simulink model "Equipe9_Simulateur_Matlab"  (R2023a)
settings: Solver=ode45  StartTime=0.0  StopTime=temps  RelTol=1e-7  EnableMultiTasking=on
model workspace (MAT data in the model file):
  K = 0.745
  K_2 = 0.745
  K_3 = 0.854
  T = 146.07
  T_2 = 38.431
  T_3 = 20.268
values from neighbouring files (symbols this model uses):
  ampli_diff = 3.075    [interface.m]
  B = 3984    [interface.m]
  bit_adc = 10    [interface.m]
  bit_dac = 10    [interface.m]
  courant_finale = 1    [interface.m]
  courant_initiale = 0    [interface.m]
  courant_timer = 10    [interface.m]
  Cte_filtre = 0.00944    [interface.m]
  Cte_perturbation = 150.4664    [interface.m]
  Cte_perturbationT2 = 150.3737    [interface.m]
  Cte_T1 = 90.126    [interface.m]
  Cte_T2 = 38.431    [interface.m]
  Cte_T3 = 20.268    [interface.m]
  final_temps = temps    (= 1000)    [interface.m]
  finalPower = 0    [interface.m]
  finalTemp = 25    [interface.m]
  Gain_circuit_sortie = 0.24801    [interface.m]
  Gain_perturbation = 6.1526    [interface.m]
  Gain_perturbationT2 = 5.5789    [interface.m]
  Gain_puissance = 3.2071    [interface.m]
  Gain_T1 = 8.192    [interface.m]
  Gain_T2 = 0.745    [interface.m]
  Gain_T3 = 0.854    [interface.m]
  gainReg = 0.1    [interface.m]
  initialPower = 0    [interface.m]
  initialTemp = 23    [interface.m]
  initialTime = 0    [interface.m]
  plus_petite = 1.735    [interface.m]
  ProportionT2 = 1    [interface.m]
  R_0 = 10000    [interface.m]
  samplingTime = 3    [interface.m]
  T_0 = 298.15    [interface.m]
  tempsReg = 130    [interface.m]
  V_ref = 2.521    [interface.m]
  variance = 0.0025    [interface.m]
undefined symbols (not defined in the file or in its folder): boucleouverte, pwm_ouvert, samplingTimePWM
libraries: eePwmGenerator x1
settings Model: Creator=LiberT  LastModifiedBy=SAPAR95
settings SolverCC: AlgebraicLoopSolver=TrustRegion
settings DataIOCC: LimitDataPoints=on  SaveFormat=Array  SignalLoggingSaveFormat=ModelDataLogs  ReturnWorkspaceOutputs=off
settings OptimizationCC: BlockReduction=off  BooleanDataType=off  OptimizeBlockIOStorage=off  ExpressionDepthLimit=2147483647  InitFltsAndDblsToZero=on  LifeSpan=inf
settings DebuggingCC: SaveWithParameterizedLinksMsg=none  UnderspecifiedInitializationDetection=Classic  MergeDetectMultiDrivingBlocksExec=none  SignalResolutionControl=TryResolveAllWithWarning  MultiTaskDSMMsg=warning  MultiTaskCondExecSysMsg=none  FcnCallInpInsideContextMsg=warning  UnconnectedInputMsg=warning  UnconnectedOutputMsg=warning  UnconnectedLineMsg=warning  StateNameClashWarn=warning  SFUnexpectedBacktrackingDiag=warning  SFNoUnconditionalDefaultTransitionDiag=warning  SFExecutionAtInitializationDiag=none  ArithmeticOperatorsInVariantConditions=warning
settings HardwareCC: ProdBitPerPointer=32  ProdBitPerSizeT=32  ProdBitPerPtrDiffT=32  ProdLargestAtomicFloat=None  ProdIntDivRoundTo=Undefined  ProdEndianess=Unspecified  ProdWordSize=32  ProdHWDeviceType=32-bit Generic  TargetBitPerPointer=64  TargetBitPerSizeT=64  TargetBitPerPtrDiffT=64  TargetLongLongMode=on  TargetIntDivRoundTo=Zero  TargetEndianess=LittleEndian  TargetWordSize=64  TargetHWDeviceType=MATLAB Host  ProdEqTarget=off
settings ModelReferenceCC: EnableRefExpFcnMdlSchedulingChecks=on  PropagateSignalLabelsOutOfModel=off
settings SFSimCC: SimUseLocalCustomCode=off  CustomCodeUndefinedFunction=UseInterfaceOnly
settings RTWCC: RTWUseLocalCustomCode=off
settings CodeAppCC: StateflowObjectComments=on
settings GRTTargetCC: TargetFcnLib=ansi_tfl_tmw.mat  TargetLangStandard=C89/C90 (ANSI)  ModelReferenceCompliant=off  CompOptLevelCompliant=off  CombineOutputUpdateFcns=off  MatFileLogging=off  GRTInterface=on
settings ConfigComp: CovMetricSettings=dw  CovSaveCumulativeToWorkspaceVar=on  CovSaveSingleToWorkspaceVar=on  CovExternalEMLEnable=off

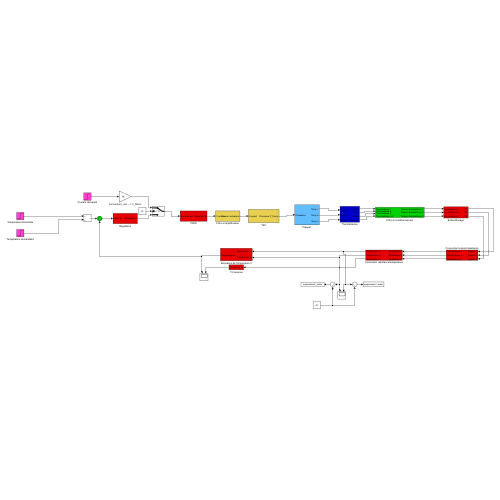
[thumbnail: Simulink's stored preview of the top-level diagram]
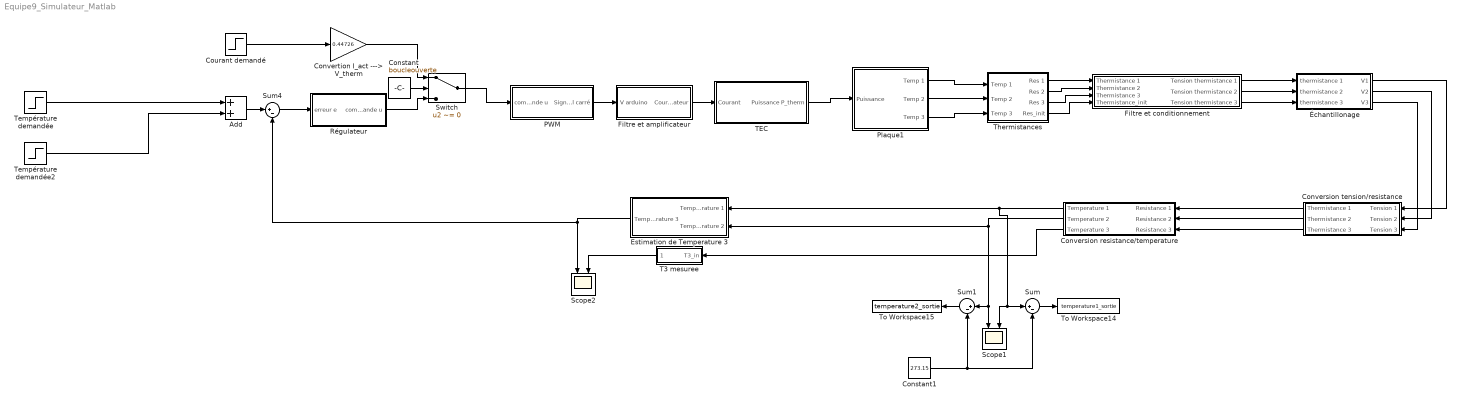
== system Equipe9_Simulateur_Matlab ==
  Add : Sum
  Constant : Constant  Value=boucleouverte
  Constant1 : Constant  Value=273.15
  Conversion resistance/temperature : Subsystem
  Conversion tension/resistance : Subsystem
  Convertion I_act ---> V_therm : Gain  Gain=0.44726
  Courant demandé : Step  Time=courant_timer  Before=courant_initiale  After=courant_finale  SampleTime=0
  Estimation de Temperature 3 : Subsystem
  Filtre et amplificateur : Subsystem
  Filtre et conditionnement : Subsystem
  PWM : Subsystem
  Plaque1 : Subsystem
  Régulateur : Subsystem
  Scope1 : Scope  NumInputPorts=2
  Scope2 : Scope  NumInputPorts=2
  Sum : Sum  Inputs=|+-
  Sum1 : Sum  Inputs=|+-
  Sum4 : Sum  Inputs=|+-  InputSameDT=on  SaturateOnIntegerOverflow=on  OutDataTypeStr=Inherit: Same as first input
  Switch : Switch  Criteria=u2 ~= 0  Threshold=false  SaturateOnIntegerOverflow=off  InputSameDT=off
  T3 mesuree : Subsystem
  TEC : Subsystem
  Température demandée : Step  Time=0  Before=initialTemp  After=finalTemp  SampleTime=0
  Température demandée2 : Step  Time=final_temps  After=final_final-finalTemp  SampleTime=0
  Thermistances : Subsystem
  To Workspace14 : ToWorkspace  VariableName=temperature1_sortie  SaveFormat=Timeseries  SampleTime=samplingTime
  To Workspace15 : ToWorkspace  VariableName=temperature2_sortie  SaveFormat=Timeseries  SampleTime=samplingTime
  Échantillonage : Subsystem
  wires:
  Sum4/1 -> Régulateur/1(erreur e)
  Plaque1/3(Temp 3) -> Thermistances/3(Temp 3)
  Filtre et amplificateur/1(Courant actuateur) -> TEC/1(Courant)
  Plaque1/1(Temp 1) -> Thermistances/1(Temp 1)
  Plaque1/2(Temp 2) -> Thermistances/2(Temp 2)
  Filtre et conditionnement/1(Tension thermistance 1) -> Échantillonage/1(thermistance 1)
  Conversion tension/resistance/2(Thermistance 2) -> Conversion resistance/temperature/2(Resistance 2)
  Conversion resistance/temperature/1(Temperature 1) -> Sum/1, Scope1/2, Estimation de Temperature 3/1(Temperature 1)
  Conversion resistance/temperature/2(Temperature 2) -> Sum1/1, Scope1/1, Estimation de Temperature 3/2(Temperature 2)
  Estimation de Temperature 3/1(Temperature 3) -> Scope2/1, Sum4/2
  PWM/1(Signal carré) -> Filtre et amplificateur/1(V arduino)
  Thermistances/3(Res 3) -> Filtre et conditionnement/3(Thermistance 3)
  Thermistances/2(Res 2) -> Filtre et conditionnement/2(Thermistance 2)
  T3 mesuree/1(T3_out) -> Scope2/2
  Conversion resistance/temperature/3(Temperature 3) -> T3 mesuree/1(T3_in)
  Filtre et conditionnement/3(Tension thermistance 3) -> Échantillonage/3(thermistance 3)
  Échantillonage/1(V1) -> Conversion tension/resistance/1(Tension 1)
  Échantillonage/2(V2) -> Conversion tension/resistance/2(Tension 2)
  Échantillonage/3(V3) -> Conversion tension/resistance/3(Tension 3)
  Régulateur/1(commande u) -> Switch/3
  Switch/1 -> PWM/1(commande u)
  Constant/1 -> Switch/2
  Courant demandé/1 -> Convertion I_act ---> V_therm/1
  Convertion I_act ---> V_therm/1 -> Switch/1
  Thermistances/1(Res 1) -> Filtre et conditionnement/1(Thermistance 1)
  Conversion tension/resistance/3(Thermistance 3) -> Conversion resistance/temperature/3(Resistance 3)
  Conversion tension/resistance/1(Thermistance 1) -> Conversion resistance/temperature/1(Resistance 1)
  Filtre et conditionnement/2(Tension thermistance 2) -> Échantillonage/2(thermistance 2)
  TEC/1(Puissance P_therm) -> Plaque1/1(Puissance)
  Thermistances/4(Res_init) -> Filtre et conditionnement/4(Thermistance_init)
  Température demandée/1 -> Add/1
  Température demandée2/1 -> Add/2
  Add/1 -> Sum4/1
  Sum/1 -> To Workspace14/1
  Constant1/1 -> Sum1/2, Sum/2
  Sum1/1 -> To Workspace15/1

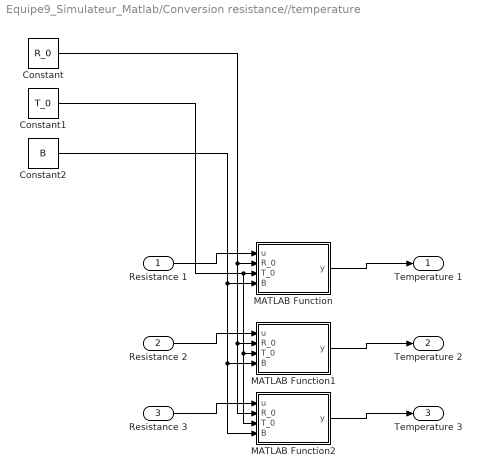
== system Equipe9_Simulateur_Matlab/Conversion resistance//temperature ==
  Resistance 1 : Inport
  Resistance 2 : Inport  Port=2
  Resistance 3 : Inport  Port=3
  Constant : Constant  Value=R_0
  Constant1 : Constant  Value=T_0
  Constant2 : Constant  Value=B
  MATLAB Function : MATLAB Function  TreatAsAtomicUnit=on
  MATLAB Function1 : MATLAB Function  TreatAsAtomicUnit=on
  MATLAB Function2 : MATLAB Function  TreatAsAtomicUnit=on
  Temperature 1 : Outport
  Temperature 2 : Outport  Port=2
  Temperature 3 : Outport  Port=3
  wires:
  Resistance 1/1 -> MATLAB Function/1(u)
  MATLAB Function/1(y) -> Temperature 1/1
  Resistance 2/1 -> MATLAB Function1/1(u)
  MATLAB Function1/1(y) -> Temperature 2/1
  Resistance 3/1 -> MATLAB Function2/1(u)
  MATLAB Function2/1(y) -> Temperature 3/1
  Constant/1 -> MATLAB Function2/2(R_0), MATLAB Function1/2(R_0), MATLAB Function/2(R_0)
  Constant1/1 -> MATLAB Function2/3(T_0), MATLAB Function1/3(T_0), MATLAB Function/3(T_0)
  Constant2/1 -> MATLAB Function/4(B), MATLAB Function1/4(B), MATLAB Function2/4(B)

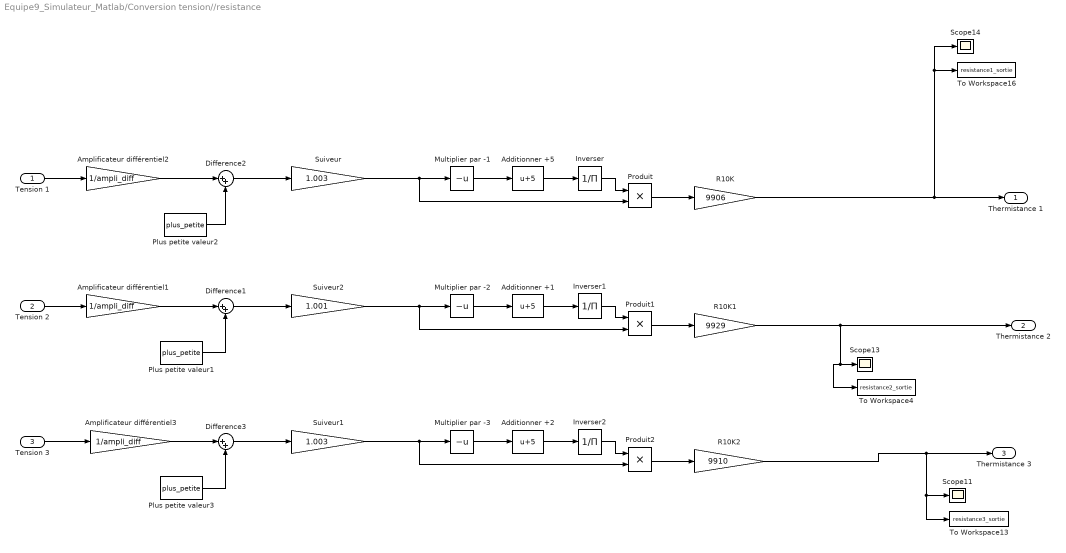
== system Equipe9_Simulateur_Matlab/Conversion tension//resistance ==
  Tension 1 : Inport
  Tension 2 : Inport  Port=2
  Tension 3 : Inport  Port=3
  Additionner +1 : Bias  Bias=5  SaturateOnIntegerOverflow=off
  Additionner +2 : Bias  Bias=5  SaturateOnIntegerOverflow=off
  Additionner +5 : Bias  Bias=5  SaturateOnIntegerOverflow=off
  Amplificateur différentiel1 : Gain  Gain=1/ampli_diff
  Amplificateur différentiel2 : Gain  Gain=1/ampli_diff
  Amplificateur différentiel3 : Gain  Gain=1/ampli_diff
  Difference1 : Sum  Inputs=|++
  Difference2 : Sum  Inputs=|++
  Difference3 : Sum  Inputs=|++
  Inverser : Product  Inputs=/
  Inverser1 : Product  Inputs=/
  Inverser2 : Product  Inputs=/
  Multiplier par -1 : UnaryMinus
  Multiplier par -2 : UnaryMinus
  Multiplier par -3 : UnaryMinus
  Plus petite valeur1 : Constant  Value=plus_petite
  Plus petite valeur2 : Constant  Value=plus_petite
  Plus petite valeur3 : Constant  Value=plus_petite
  Produit : Product
  Produit1 : Product
  Produit2 : Product
  R10K : Gain  Gain=9906
  R10K1 : Gain  Gain=9929
  R10K2 : Gain  Gain=9910
  Scope11 : Scope
  Scope13 : Scope
  Scope14 : Scope
  Suiveur : Gain  Gain=1.003
  Suiveur1 : Gain  Gain=1.003
  Suiveur2 : Gain  Gain=1.001
  To Workspace13 : ToWorkspace  VariableName=resistance3_sortie  SaveFormat=Timeseries  SampleTime=samplingTime
  To Workspace16 : ToWorkspace  VariableName=resistance1_sortie  SaveFormat=Timeseries  SampleTime=samplingTime
  To Workspace4 : ToWorkspace  VariableName=resistance2_sortie  SaveFormat=Timeseries  SampleTime=samplingTime
  Thermistance 1 : Outport
  Thermistance 2 : Outport  Port=2
  Thermistance 3 : Outport  Port=3
  wires:
  Difference2/1 -> Suiveur/1
  Inverser/1 -> Produit/1
  Multiplier par -1/1 -> Additionner +5/1
  Produit/1 -> R10K/1
  Additionner +5/1 -> Inverser/1
  Amplificateur différentiel2/1 -> Difference2/1
  Plus petite valeur2/1 -> Difference2/2
  Tension 1/1 -> Amplificateur différentiel2/1
  Plus petite valeur1/1 -> Difference1/2
  Difference1/1 -> Suiveur2/1
  Produit1/1 -> R10K1/1
  Tension 2/1 -> Amplificateur différentiel1/1
  Amplificateur différentiel1/1 -> Difference1/1
  Multiplier par -2/1 -> Additionner +1/1
  Inverser1/1 -> Produit1/1
  Additionner +1/1 -> Inverser1/1
  Additionner +2/1 -> Inverser2/1
  Multiplier par -3/1 -> Additionner +2/1
  Amplificateur différentiel3/1 -> Difference3/1
  Plus petite valeur3/1 -> Difference3/2
  Inverser2/1 -> Produit2/1
  Difference3/1 -> Suiveur1/1
  Tension 3/1 -> Amplificateur différentiel3/1
  Produit2/1 -> R10K2/1
  Suiveur/1 -> Produit/2, Multiplier par -1/1
  Suiveur1/1 -> Produit2/2, Multiplier par -3/1
  Suiveur2/1 -> Produit1/2, Multiplier par -2/1
  R10K/1 -> Scope14/1, To Workspace16/1, Thermistance 1/1
  R10K1/1 -> To Workspace4/1, Scope13/1, Thermistance 2/1
  R10K2/1 -> To Workspace13/1, Scope11/1, Thermistance 3/1

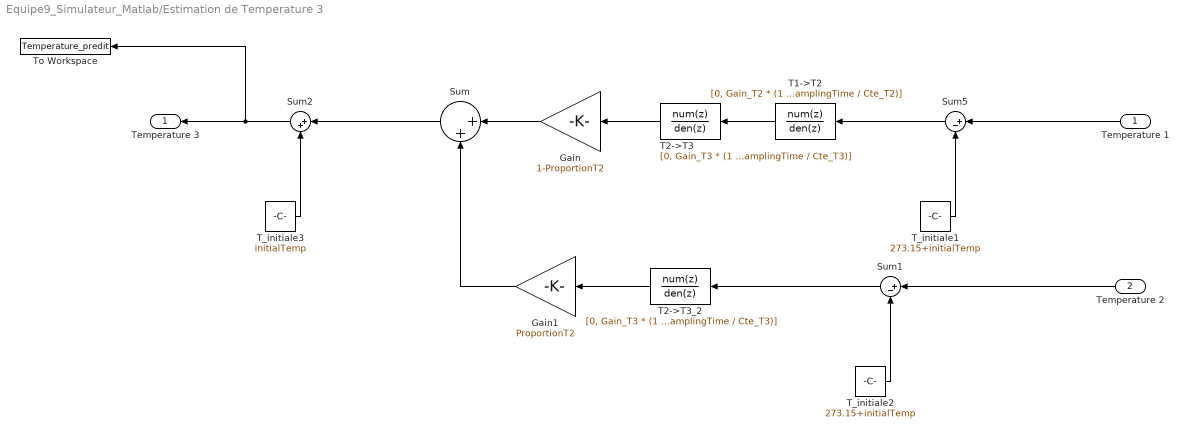
== system Equipe9_Simulateur_Matlab/Estimation de Temperature 3 ==
  Temperature 1 : Inport
  Temperature 2 : Inport  Port=2
  Gain : Gain  Gain=1-ProportionT2
  Gain1 : Gain  Gain=ProportionT2
  Sum : Sum  Inputs=|++
  Sum1 : Sum  Inputs=|+-  InputSameDT=on  SaturateOnIntegerOverflow=on  OutDataTypeStr=Inherit: Same as first input
  Sum2 : Sum  Inputs=|++  InputSameDT=on  SaturateOnIntegerOverflow=on  OutDataTypeStr=Inherit: Same as first input
  Sum5 : Sum  Inputs=|+-  InputSameDT=on  SaturateOnIntegerOverflow=on  OutDataTypeStr=Inherit: Same as first input
  T1->T2 : DiscreteFilter  Numerator=[0, Gain_T2 * (1 - exp(-samplingTime / Cte_T2))]  Denominator=[1, -exp(-samplingTime / Cte_T2)]  SampleTime=samplingTime
  T2->T3 : DiscreteFilter  Numerator=[0, Gain_T3 * (1 - exp(-samplingTime / Cte_T3))]  Denominator=[1, -exp(-samplingTime / Cte_T3)]  SampleTime=samplingTime
  T2->T3_2 : DiscreteFilter  Numerator=[0, Gain_T3 * (1 - exp(-samplingTime / Cte_T3))]  Denominator=[1, -exp(-samplingTime / Cte_T3)]  SampleTime=samplingTime
  T_initiale1 : Constant  Value=273.15+initialTemp
  T_initiale2 : Constant  Value=273.15+initialTemp
  T_initiale3 : Constant  Value=initialTemp
  To Workspace : ToWorkspace  VariableName=Temperature_predit  SaveFormat=Timeseries  SampleTime=samplingTime
  Temperature 3 : Outport
  wires:
  Temperature 2/1 -> Sum1/1
  T_initiale2/1 -> Sum1/2
  T_initiale3/1 -> Sum2/2
  Sum1/1 -> T2->T3_2/1
  T1->T2/1 -> T2->T3/1
  T2->T3/1 -> Gain/1
  Sum5/1 -> T1->T2/1
  Temperature 1/1 -> Sum5/1
  T_initiale1/1 -> Sum5/2
  Sum/1 -> Sum2/1
  T2->T3_2/1 -> Gain1/1
  Gain/1 -> Sum/1
  Gain1/1 -> Sum/2
  Sum2/1 -> To Workspace/1, Temperature 3/1

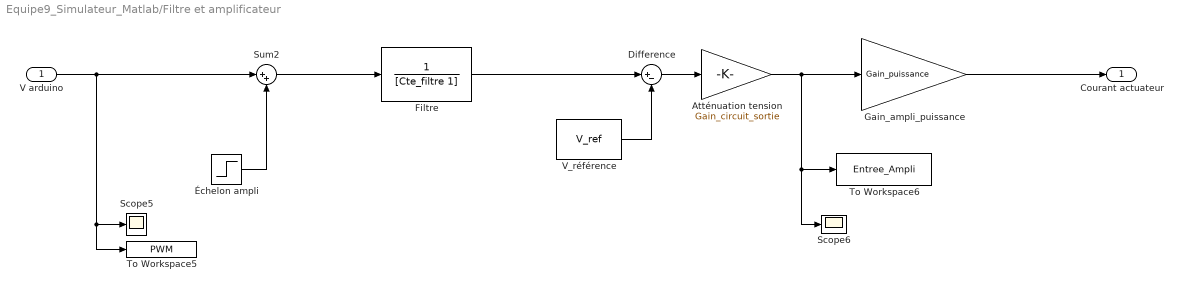
== system Equipe9_Simulateur_Matlab/Filtre et amplificateur ==
  V arduino : Inport
  Atténuation tension : Gain  Gain=Gain_circuit_sortie
  Difference : Sum  Inputs=|+-
  Filtre : TransferFcn  Numerator=1  Denominator=[Cte_filtre 1]
  Gain_ampli_puissance : Gain  Gain=Gain_puissance
  Scope5 : Scope
  Scope6 : Scope
  Sum2 : Sum  Inputs=|++  InputSameDT=on  SaturateOnIntegerOverflow=on  OutDataTypeStr=Inherit: Same as first input
  To Workspace5 : ToWorkspace  VariableName=PWM  SaveFormat=Timeseries  SampleTime=samplingTime
  To Workspace6 : ToWorkspace  VariableName=Entree_Ampli  SaveFormat=Timeseries  SampleTime=samplingTime
  V_référence : Constant  Value=V_ref
  "Échelon ampli " : Step  Time=0  After=0  SampleTime=samplingTime
  Courant actuateur : Outport
  wires:
  V_référence/1 -> Difference/2
  Difference/1 -> Atténuation tension/1
  Sum2/1 -> Filtre/1
  "Échelon ampli "/1 -> Sum2/2
  Filtre/1 -> Difference/1
  Atténuation tension/1 -> Scope6/1, To Workspace6/1, Gain_ampli_puissance/1
  Gain_ampli_puissance/1 -> Courant actuateur/1
  V arduino/1 -> To Workspace5/1, Scope5/1, Sum2/1

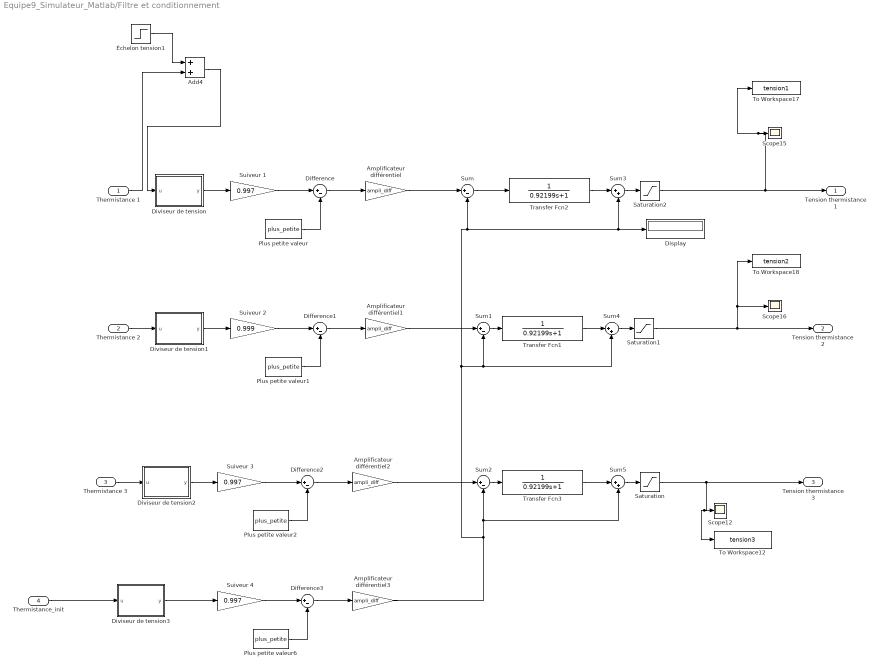
== system Equipe9_Simulateur_Matlab/Filtre et conditionnement ==
  Thermistance 1 : Inport
  Thermistance 2 : Inport  Port=2
  Thermistance 3 : Inport  Port=3
  Thermistance_init : Inport  Port=4
  Add4 : Sum
  Amplificateur différentiel{,1..3} (4 alike) : Gain  Gain=ampli_diff
  Difference{,1..3} (4 alike) : Sum  Inputs=|+-
  Display : Display
  Diviseur de tension : MATLAB Function  TreatAsAtomicUnit=on
  Diviseur de tension1 : MATLAB Function  TreatAsAtomicUnit=on
  Diviseur de tension2 : MATLAB Function  TreatAsAtomicUnit=on
  Diviseur de tension3 : MATLAB Function  TreatAsAtomicUnit=on
  Plus petite valeur{,1..2,6} (4 alike) : Constant  Value=plus_petite
  Saturation : Saturate  UpperLimit=5  LowerLimit=0
  Saturation1 : Saturate  UpperLimit=5  LowerLimit=0
  Saturation2 : Saturate  UpperLimit=4.5  LowerLimit=0
  Scope12 : Scope
  Scope15 : Scope
  Scope16 : Scope
  Suiveur 1 : Gain  Gain=0.997
  Suiveur 2 : Gain  Gain=0.999
  Suiveur 3 : Gain  Gain=0.997
  Suiveur 4 : Gain  Gain=0.997
  Sum : Sum  Inputs=|+-
  Sum1 : Sum  Inputs=|+-
  Sum2 : Sum  Inputs=|+-
  Sum3 : Sum  Inputs=|++
  Sum4 : Sum  Inputs=|++
  Sum5 : Sum  Inputs=|++
  To Workspace12 : ToWorkspace  VariableName=tension3  SaveFormat=Timeseries  SampleTime=samplingTime
  To Workspace17 : ToWorkspace  VariableName=tension1  SaveFormat=Timeseries  SampleTime=samplingTime
  To Workspace18 : ToWorkspace  VariableName=tension2  SaveFormat=Timeseries  SampleTime=samplingTime
  Transfer Fcn1 : TransferFcn  Denominator=[0.92199 1]
  Transfer Fcn2 : TransferFcn  Denominator=[0.92199 1]
  Transfer Fcn3 : TransferFcn  Denominator=[0.92199 1]
  Échelon tension1 : Step  Time=0  After=0  SampleTime=samplingTime
  Tension thermistance 1 : Outport
  Tension thermistance 2 : Outport  Port=2
  Tension thermistance 3 : Outport  Port=3
  wires:
  Difference/1 -> Amplificateur différentiel/1
  Diviseur de tension/1(y) -> Suiveur 1/1
  Plus petite valeur/1 -> Difference/2
  Suiveur 1/1 -> Difference/1
  Plus petite valeur1/1 -> Difference1/2
  Difference1/1 -> Amplificateur différentiel1/1
  Diviseur de tension1/1(y) -> Suiveur 2/1
  Suiveur 2/1 -> Difference1/1
  Thermistance 2/1 -> Diviseur de tension1/1(u)
  Suiveur 3/1 -> Difference2/1
  Plus petite valeur2/1 -> Difference2/2
  Thermistance 3/1 -> Diviseur de tension2/1(u)
  Diviseur de tension2/1(y) -> Suiveur 3/1
  Difference2/1 -> Amplificateur différentiel2/1
  Sum/1 -> Transfer Fcn2/1
  Sum1/1 -> Transfer Fcn1/1
  Sum2/1 -> Transfer Fcn3/1
  Amplificateur différentiel/1 -> Sum/1
  Transfer Fcn2/1 -> Sum3/1
  Amplificateur différentiel1/1 -> Sum1/1
  Transfer Fcn1/1 -> Sum4/1
  Amplificateur différentiel2/1 -> Sum2/1
  Transfer Fcn3/1 -> Sum5/1
  Échelon tension1/1 -> Add4/1
  Thermistance 1/1 -> Add4/2
  Add4/1 -> Diviseur de tension/1(u)
  Amplificateur différentiel3/1 -> Display/1, Sum3/2, Sum/2, Sum4/2, Sum1/2, Sum5/2, Sum2/2
  Difference3/1 -> Amplificateur différentiel3/1
  Diviseur de tension3/1(y) -> Suiveur 4/1
  Plus petite valeur6/1 -> Difference3/2
  Suiveur 4/1 -> Difference3/1
  Thermistance_init/1 -> Diviseur de tension3/1(u)
  Sum5/1 -> Saturation/1
  Sum4/1 -> Saturation1/1
  Sum3/1 -> Saturation2/1
  Saturation/1 -> To Workspace12/1, Scope12/1, Tension thermistance 3/1
  Saturation2/1 -> To Workspace17/1, Scope15/1, Tension thermistance 1/1
  Saturation1/1 -> Scope16/1, To Workspace18/1, Tension thermistance 2/1

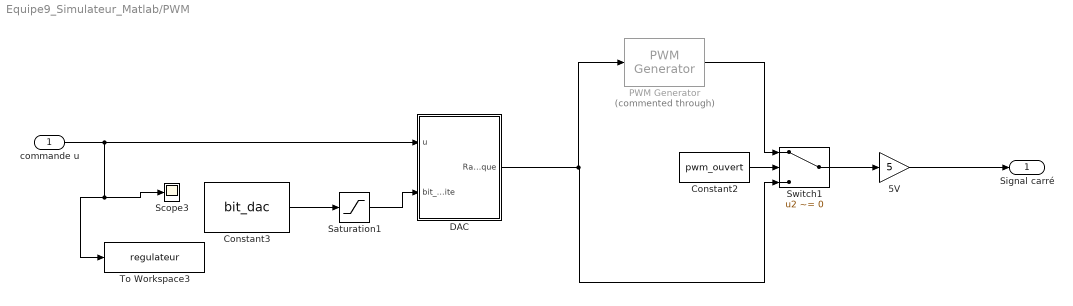
== system Equipe9_Simulateur_Matlab/PWM ==
  commande u : Inport
  5V : Gain  Gain=5
  Constant2 : Constant  Value=pwm_ouvert
  Constant3 : Constant  Value=bit_dac
  DAC : MATLAB Function  TreatAsAtomicUnit=on
  PWM Generator : eePwmGenerator/PWM Generator  Commented=through  CarrCount=Up  Tper=1023*10^-6  Tdelay=0  Ts=(1023*10^-6)/((2^samplingTimePWM)-1)
  Saturation1 : Saturate  UpperLimit=16  LowerLimit=1
  Scope3 : Scope
  Switch1 : Switch  Criteria=u2 ~= 0  Threshold=false  SaturateOnIntegerOverflow=off  InputSameDT=off
  To Workspace3 : ToWorkspace  VariableName=regulateur  SaveFormat=Timeseries  SampleTime=samplingTime
  Signal carré : Outport
  wires:
  5V/1 -> Signal carré/1
  Saturation1/1 -> DAC/2(bit_dac_limite)
  Switch1/1 -> 5V/1
  PWM Generator/1 -> Switch1/1
  DAC/1(Rapport_cyclique) -> PWM Generator/1, Switch1/3
  Constant3/1 -> Saturation1/1
  Constant2/1 -> Switch1/2
  commande u/1 -> DAC/1(u), Scope3/1, To Workspace3/1

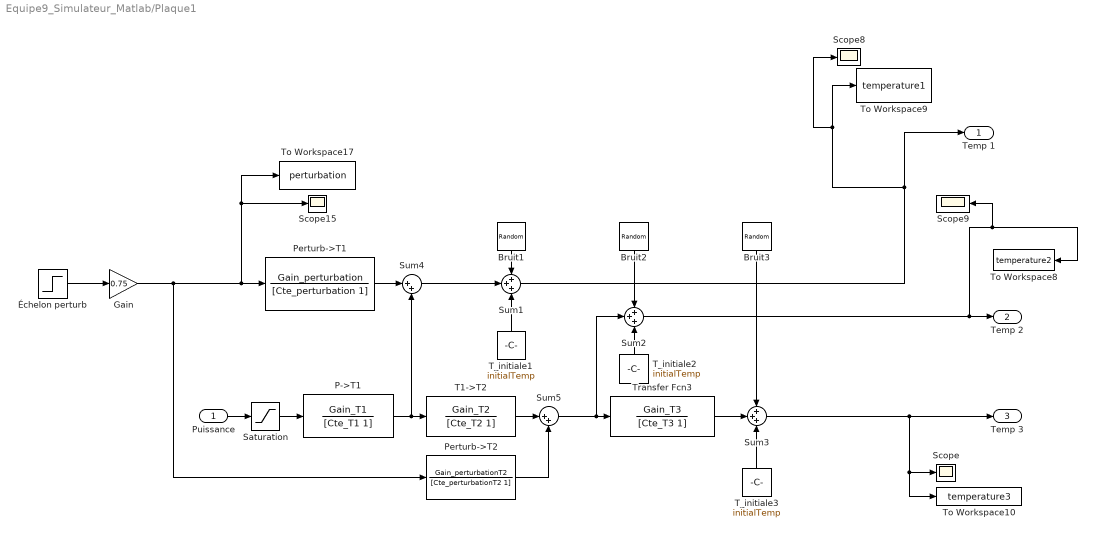
== system Equipe9_Simulateur_Matlab/Plaque1 ==
  Puissance : Inport
  Bruit1 : RandomNumber  Variance=variance  SampleTime=samplingTime
  Bruit2 : RandomNumber  Variance=variance  SampleTime=samplingTime
  Bruit3 : RandomNumber  Variance=variance  SampleTime=samplingTime
  Gain : Gain  Gain=0.75
  P->T1 : TransferFcn  Numerator=Gain_T1  Denominator=[Cte_T1 1]
  Perturb->T1 : TransferFcn  Numerator=Gain_perturbation  Denominator=[Cte_perturbation 1]
  Perturb->T2 : TransferFcn  Numerator=Gain_perturbationT2  Denominator=[Cte_perturbationT2 1]
  Saturation : Saturate  UpperLimit=3.6  LowerLimit=-2.1
  Scope{,8..9,15} (4 alike) : Scope
  Sum1 : Sum  Inputs=+++  InputSameDT=on  SaturateOnIntegerOverflow=on  OutDataTypeStr=Inherit: Same as first input
  Sum2 : Sum  Inputs=+++  InputSameDT=on  SaturateOnIntegerOverflow=on  OutDataTypeStr=Inherit: Same as first input
  Sum3 : Sum  Inputs=+++  InputSameDT=on  SaturateOnIntegerOverflow=on  OutDataTypeStr=Inherit: Same as first input
  Sum4 : Sum  Inputs=|++  InputSameDT=on  SaturateOnIntegerOverflow=on  OutDataTypeStr=Inherit: Same as first input
  Sum5 : Sum  Inputs=|++  InputSameDT=on  SaturateOnIntegerOverflow=on  OutDataTypeStr=Inherit: Same as first input
  T1->T2 : TransferFcn  Numerator=Gain_T2  Denominator=[Cte_T2 1]
  T_initiale1 : Constant  Value=initialTemp
  T_initiale2 : Constant  Value=initialTemp
  T_initiale3 : Constant  Value=initialTemp
  To Workspace10 : ToWorkspace  VariableName=temperature3  SaveFormat=Timeseries  SampleTime=samplingTime
  To Workspace17 : ToWorkspace  VariableName=perturbation  SaveFormat=Timeseries  SampleTime=samplingTime
  To Workspace8 : ToWorkspace  VariableName=temperature2  SaveFormat=Timeseries  SampleTime=samplingTime
  To Workspace9 : ToWorkspace  VariableName=temperature1  SaveFormat=Timeseries  SampleTime=samplingTime
  Transfer Fcn3 : TransferFcn  Numerator=Gain_T3  Denominator=[Cte_T3 1]
  Échelon perturb : Step  Time=initialTime  Before=initialPower  After=finalPower  SampleTime=samplingTime
  Temp 1 : Outport
  Temp 2 : Outport  Port=2
  Temp 3 : Outport  Port=3
  wires:
  P->T1/1 -> T1->T2/1, Sum4/2
  Perturb->T1/1 -> Sum4/1
  Gain/1 -> Perturb->T1/1, To Workspace17/1, Scope15/1, Perturb->T2/1
  T1->T2/1 -> Sum5/1
  Sum5/1 -> Sum2/2, Transfer Fcn3/1
  Perturb->T2/1 -> Sum5/2
  Saturation/1 -> P->T1/1
  Puissance/1 -> Saturation/1
  Bruit1/1 -> Sum1/1
  T_initiale1/1 -> Sum1/3
  Sum4/1 -> Sum1/2
  Transfer Fcn3/1 -> Sum3/2
  T_initiale2/1 -> Sum2/3
  Bruit2/1 -> Sum2/1
  Bruit3/1 -> Sum3/1
  T_initiale3/1 -> Sum3/3
  Échelon perturb/1 -> Gain/1
  Sum3/1 -> To Workspace10/1, Scope/1, Temp 3/1
  Sum1/1 -> Scope8/1, To Workspace9/1, Temp 1/1
  Sum2/1 -> Scope9/1, To Workspace8/1, Temp 2/1

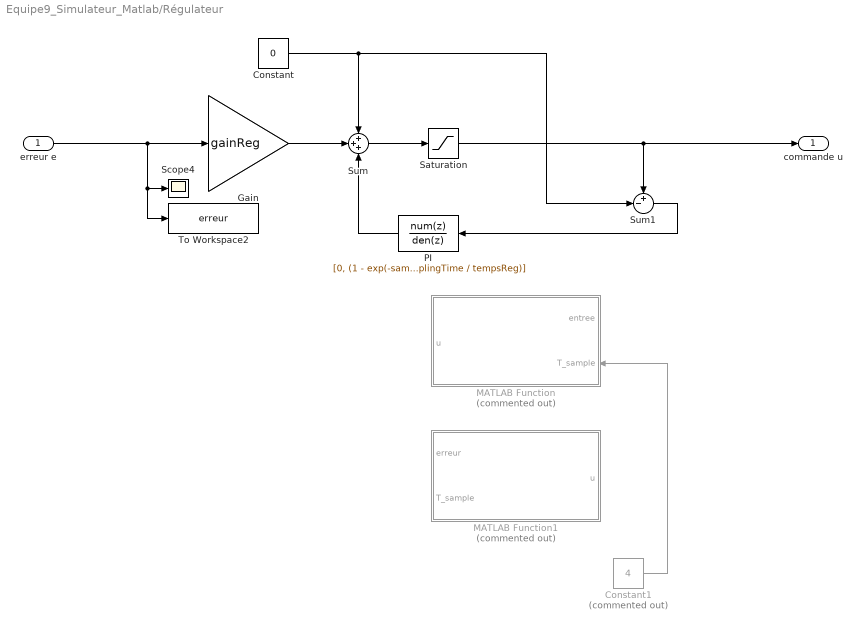
== system Equipe9_Simulateur_Matlab/Régulateur ==
  erreur e : Inport
  Constant : Constant  Value=0
  Constant1 : Constant  Commented=on  Value=4
  Gain : Gain  Gain=gainReg
  MATLAB Function : MATLAB Function  Commented=on  TreatAsAtomicUnit=on
  MATLAB Function1 : MATLAB Function  Commented=on  TreatAsAtomicUnit=on
  PI : DiscreteFilter  Numerator=[0, (1 - exp(-samplingTime / tempsReg))]  Denominator=[1, -exp(-samplingTime / tempsReg)]  SampleTime=samplingTime
  Saturation : Saturate  UpperLimit=0.9  LowerLimit=-0.9
  Scope4 : Scope
  Sum : Sum  Inputs=+++
  Sum1 : Sum  Inputs=+-|
  To Workspace2 : ToWorkspace  VariableName=erreur  SaveFormat=Timeseries  SampleTime=samplingTime
  commande u : Outport
  wires:
  Saturation/1 -> Sum1/1, commande u/1
  Gain/1 -> Sum/2
  Sum/1 -> Saturation/1
  Constant/1 -> Sum1/2, Sum/1
  Sum1/1 -> PI/1
  PI/1 -> Sum/3
  Constant1/1 -> MATLAB Function/2(T_sample)
  erreur e/1 -> To Workspace2/1, Scope4/1, Gain/1

== system Equipe9_Simulateur_Matlab/T3 mesuree ==
  T3_in : Inport
  Sum2 : Sum  Inputs=|+-  InputSameDT=on  SaturateOnIntegerOverflow=on  OutDataTypeStr=Inherit: Same as first input
  T_initiale1 : Constant  Value=273.15
  To Workspace1 : ToWorkspace  VariableName=Temperature_simulation  SaveFormat=Timeseries  SampleTime=samplingTime
  T3_out : Outport
  wires:
  T_initiale1/1 -> Sum2/2
  T3_in/1 -> Sum2/1
  Sum2/1 -> To Workspace1/1, T3_out/1

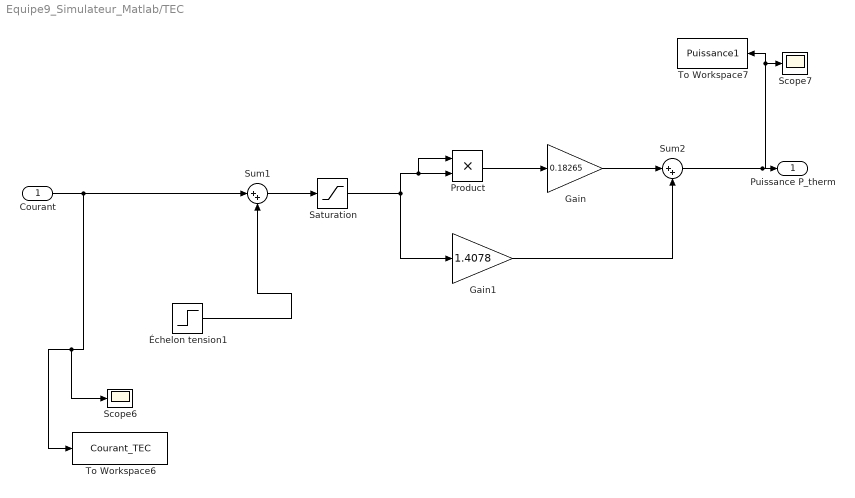
== system Equipe9_Simulateur_Matlab/TEC ==
  Courant : Inport
  Gain : Gain  Gain=0.18265
  Gain1 : Gain  Gain=1.4078
  Product : Product
  Saturation : Saturate  UpperLimit=2.00292  LowerLimit=-2.02152
  Scope6 : Scope
  Scope7 : Scope
  Sum1 : Sum  Inputs=|++  InputSameDT=on  SaturateOnIntegerOverflow=on  OutDataTypeStr=Inherit: Same as first input
  Sum2 : Sum  Inputs=|++  InputSameDT=on  SaturateOnIntegerOverflow=on  OutDataTypeStr=Inherit: Same as first input
  To Workspace6 : ToWorkspace  VariableName=Courant_TEC  SaveFormat=Timeseries  SampleTime=samplingTime
  To Workspace7 : ToWorkspace  VariableName=Puissance1  SaveFormat=Timeseries  SampleTime=samplingTime
  Échelon tension1 : Step  Time=0  After=0  SampleTime=samplingTime
  Puissance P_therm : Outport
  wires:
  Échelon tension1/1 -> Sum1/2
  Product/1 -> Gain/1
  Gain/1 -> Sum2/1
  Gain1/1 -> Sum2/2
  Saturation/1 -> Product/1, Product/2, Gain1/1
  Sum1/1 -> Saturation/1
  Courant/1 -> Scope6/1, To Workspace6/1, Sum1/1
  Sum2/1 -> To Workspace7/1, Scope7/1, Puissance P_therm/1

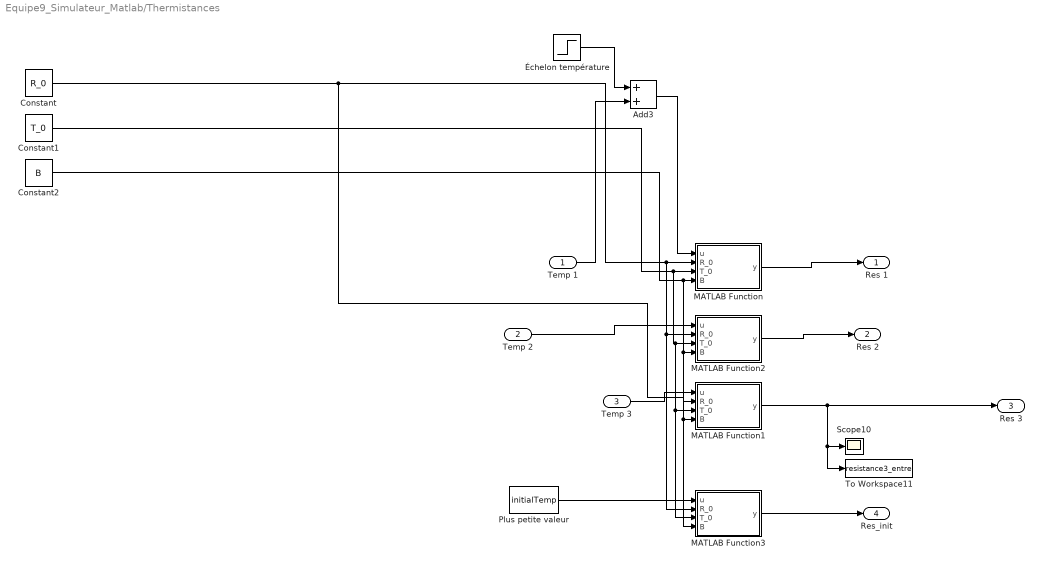
== system Equipe9_Simulateur_Matlab/Thermistances ==
  Temp 1 : Inport
  Temp 2 : Inport  Port=2
  Temp 3 : Inport  Port=3
  Add3 : Sum
  Constant : Constant  Value=R_0
  Constant1 : Constant  Value=T_0
  Constant2 : Constant  Value=B
  MATLAB Function : MATLAB Function  TreatAsAtomicUnit=on
  MATLAB Function1 : MATLAB Function  TreatAsAtomicUnit=on
  MATLAB Function2 : MATLAB Function  TreatAsAtomicUnit=on
  MATLAB Function3 : MATLAB Function  TreatAsAtomicUnit=on
  Plus petite valeur : Constant  Value=initialTemp
  Scope10 : Scope
  To Workspace11 : ToWorkspace  VariableName=resistance3_entre  SaveFormat=Timeseries  SampleTime=samplingTime
  Échelon température : Step  Time=0  After=0  SampleTime=samplingTime
  Res 1 : Outport
  Res 2 : Outport  Port=2
  Res 3 : Outport  Port=3
  Res_init : Outport  Port=4
  wires:
  MATLAB Function/1(y) -> Res 1/1
  Temp 2/1 -> MATLAB Function2/1(u)
  MATLAB Function2/1(y) -> Res 2/1
  Temp 3/1 -> MATLAB Function1/1(u)
  Échelon température/1 -> Add3/1
  Temp 1/1 -> Add3/2
  Add3/1 -> MATLAB Function/1(u)
  Constant/1 -> MATLAB Function1/2(R_0), MATLAB Function/2(R_0), MATLAB Function3/2(R_0), MATLAB Function2/2(R_0)
  Constant1/1 -> MATLAB Function2/3(T_0), MATLAB Function3/3(T_0), MATLAB Function1/3(T_0), MATLAB Function/3(T_0)
  MATLAB Function3/1(y) -> Res_init/1
  Constant2/1 -> MATLAB Function3/4(B), MATLAB Function1/4(B), MATLAB Function2/4(B), MATLAB Function/4(B)
  Plus petite valeur/1 -> MATLAB Function3/1(u)
  MATLAB Function1/1(y) -> Res 3/1, To Workspace11/1, Scope10/1

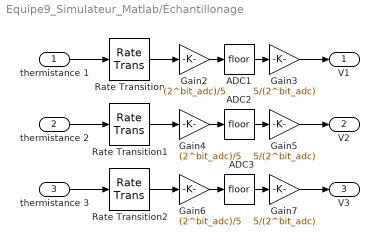
== system Equipe9_Simulateur_Matlab/Échantillonage ==
  thermistance 1 : Inport
  thermistance 2 : Inport  Port=2
  thermistance 3 : Inport  Port=3
  ADC1 : Rounding
  ADC2 : Rounding
  ADC3 : Rounding
  Gain2 : Gain  Gain=(2^bit_adc)/5
  Gain3 : Gain  Gain=5/(2^bit_adc)
  Gain4 : Gain  Gain=(2^bit_adc)/5
  Gain5 : Gain  Gain=5/(2^bit_adc)
  Gain6 : Gain  Gain=(2^bit_adc)/5
  Gain7 : Gain  Gain=5/(2^bit_adc)
  Rate Transition : RateTransition  OutPortSampleTime=samplingTime
  Rate Transition1 : RateTransition  OutPortSampleTime=samplingTime
  Rate Transition2 : RateTransition  OutPortSampleTime=samplingTime
  V1 : Outport
  V2 : Outport  Port=2
  V3 : Outport  Port=3
  wires:
  thermistance 3/1 -> Rate Transition2/1
  thermistance 1/1 -> Rate Transition/1
  thermistance 2/1 -> Rate Transition1/1
  ADC1/1 -> Gain3/1
  Gain2/1 -> ADC1/1
  ADC2/1 -> Gain5/1
  Gain4/1 -> ADC2/1
  ADC3/1 -> Gain7/1
  Gain6/1 -> ADC3/1
  Rate Transition/1 -> Gain2/1
  Gain3/1 -> V1/1
  Rate Transition1/1 -> Gain4/1
  Gain5/1 -> V2/1
  Rate Transition2/1 -> Gain6/1
  Gain7/1 -> V3/1

== matlab function Equipe9_Simulateur_Matlab/Thermistances/MATLAB Function1 ==
  data: u input; y output; R_0 input; T_0 input; B input
function y = fcn(u,R_0,T_0,B) % Fonction non linéaire
% y = R(T) = la valeur de la résistance en fonction de la température (en degré)
% u = T = La température de la plaque (en degré)


y = R_0 .* exp(B .* ((1 ./ (u+273.15)) - (1 ./ T_0)));

end

%function y = fcn(u) % Fonction d'approximation (série de Taylor)
% y = R(T) = la valeur de la résistance en fonction de la température (en degré)
% u = T = La température de la plaque (en degré)

%R0 = 10000; % Valeur de la résistance à une température de référence (25 oC = 298.15 K)
%T0 = 298.15; % Température de référence
%B = 3984; % coefficient Beta

%Gain_elec = - (B .* R0 .* exp(-B ./ T0)) ./ (T0 .^2); % Gain donnerait -0.00071 Ohm/Kelvin

%y = R0 + Gain_elec .* ((u+273.15) - T0);

%end

== matlab function Equipe9_Simulateur_Matlab/Conversion resistance//temperature/MATLAB Function1 ==
  data: u input; y output; R_0 input; T_0 input; B input
function y = fcn(u,R_0,T_0,B) % Fonction non linéaire
% u = R(T) = la valeur de la résistance en fonction de la température (en degré)
% y = T = La température de la plaque (en degré)


y = 1 ./ ( 1 ./T_0 + (1 ./B) .* log((u) ./R_0) );

end

== matlab function Equipe9_Simulateur_Matlab/Conversion resistance//temperature/MATLAB Function2 ==
  data: u input; y output; R_0 input; T_0 input; B input
function y = fcn(u,R_0,T_0,B) % Fonction non linéaire
% u = R(T) = la valeur de la résistance en fonction de la température (en degré)
% y = T = La température de la plaque (en degré)


y = 1 ./ ( 1 ./T_0 + (1 ./B) .* log((u) ./R_0) );

end

%function y = fcn(u) % Fonction d'approximation (série de Taylor)
% y = R(T) = la valeur de la résistance en fonction de la température (en degré)
% u = T = La température de la plaque (en degré)

%R0 = 10000; % Valeur de la résistance à une température de référence (25 oC = 298.15 K)
%T0 = 298.15; % Température de référence
%B = 3984; % coefficient Beta

%Gain_elec = - (B .* R0 .* exp(-B ./ T0)) ./ (T0 .^2); % Gain donnerait -0.00071 Ohm/Kelvin

%y = R0 + Gain_elec .* ((u+273.15) - T0);

%end

== matlab function Equipe9_Simulateur_Matlab/Filtre et conditionnement/Diviseur de tension2 ==
  data: u input; y output
function y = fcn(u)
    R10k = 9910;
    y= (u /(R10k+u)) * 5 ;
end

== matlab function Equipe9_Simulateur_Matlab/Thermistances/MATLAB Function2 ==
  data: u input; y output; R_0 input; T_0 input; B input
function y = fcn(u,R_0,T_0,B) % Fonction non linéaire
% y = R(T) = la valeur de la résistance en fonction de la température (en degré)
% u = T = La température de la plaque (en degré)

y = R_0 .* exp(B .* ((1 ./ (u+273.15)) - (1 ./ T_0)));

end

%function y = fcn(u) % Fonction d'approximation (série de Taylor)
% y = R(T) = la valeur de la résistance en fonction de la température (en degré)
% u = T = La température de la plaque (en degré)

%R0 = 10000; % Valeur de la résistance à une température de référence (25 oC = 298.15 K)
%T0 = 298.15; % Température de référence
%B = 3984; % coefficient Beta

%Gain_elec = - (B .* R0 .* exp(-B ./ T0)) ./ (T0 .^2); % Gain donnerait -0.00071 Ohm/Kelvin

%y = R0 + Gain_elec .* ((u+273.15) - T0);

%end

== matlab function Equipe9_Simulateur_Matlab/Thermistances/MATLAB Function3 ==
  data: u input; y output; R_0 input; T_0 input; B input
function y = fcn(u,R_0,T_0,B) % Fonction non linéaire
% y = R(T) = la valeur de la résistance en fonction de la température (en degré)
% u = T = La température de la plaque (en degré)


y = R_0 .* exp(B .* ((1 ./ (u+273.15)) - (1 ./ T_0)));

end

%function y = fcn(u) % Fonction d'approximation (série de Taylor)
% y = R(T) = la valeur de la résistance en fonction de la température (en degré)
% u = T = La température de la plaque (en degré)

%R0 = 10000; % Valeur de la résistance à une température de référence (25 oC = 298.15 K)
%T0 = 298.15; % Température de référence
%B = 3984; % coefficient Beta

%Gain_elec = - (B .* R0 .* exp(-B ./ T0)) ./ (T0 .^2); % Gain donnerait -0.00071 Ohm/Kelvin

%y = R0 + Gain_elec .* ((u+273.15) - T0);

%end

== matlab function Equipe9_Simulateur_Matlab/Thermistances/MATLAB Function ==
  data: u input; y output; R_0 input; T_0 input; B input
function y = fcn(u,R_0,T_0,B) % Fonction non linéaire
% y = R(T) = la valeur de la résistance en fonction de la température (en degré)
% u = T = La température de la plaque (en degré)

y = R_0 .* exp(B .* ((1 ./ (u+273.15)) - (1 ./ T_0)));

end

%function y = fcn(u) % Fonction d'approximation (série de Taylor)
% y = R(T) = la valeur de la résistance en fonction de la température (en degré)
% u = T = La température de la plaque (en degré)

%R0 = 10000; % Valeur de la résistance à une température de référence (25 oC = 298.15 K)
%T0 = 298.15; % Température de référence
%B = 3984; % coefficient Beta

%Gain_elec = - (B .* R0 .* exp(-B ./ T0)) ./ (T0 .^2); % Gain donnerait -0.00071 Ohm/Kelvin

%y = R0 + Gain_elec .* ((u+273.15) - T0);

%end

== matlab function Equipe9_Simulateur_Matlab/Filtre et conditionnement/Diviseur de tension ==
  data: u input; y output
function y = fcn(u)
    R10k = 9906;
    y= (u /(R10k+u)) * 5 ;
end

== matlab function Equipe9_Simulateur_Matlab/Filtre et conditionnement/Diviseur de tension3 ==
  data: u input; y output
function y = fcn(u)
    R10k = 9910;
    y= (u /(R10k+u)) * 5 ;
end

== matlab function Equipe9_Simulateur_Matlab/Régulateur/MATLAB Function1 ==
  data: erreur input; T_sample input; u output
function u = discretise_PI(erreur, T_sample)
    % Paramètres du régulateur PI
    Ti = 146.07;     % Constante d'intégration
    Kc = 0.044317;   % Gain proportionnel
    
    % Coefficients de la discrétisation (Tustin)
    num = Kc * [(1 + (T_sample/(2*Ti))), -(1 - (T_sample/(2*Ti)))];  % Numérateur
    den = [1, -1];  % Dénominateur

    % Application du régulateur sur le signal d'erreur
    u = filter(num, den, erreur);  
end

== matlab function Equipe9_Simulateur_Matlab/PWM/DAC ==
  data: u input; Rapport_cyclique output; bit_dac_limite input
function Rapport_cyclique = duty_cycle(u, bit_dac_limite)

frac = (u+0.9) / (2*0.9);
Rapport_cyclique = (floor(frac*(2^bit_dac_limite)))/2^bit_dac_limite;

end

== matlab function Equipe9_Simulateur_Matlab/Filtre et conditionnement/Diviseur de tension1 ==
  data: u input; y output
function y = fcn(u)
    R10k = 9929;
    y= (u /(R10k+u)) * 5 ;
end

== matlab function Equipe9_Simulateur_Matlab/Régulateur/MATLAB Function ==
  data: entree input; T_sample input; u output
function u = discretise_PI(entree, T_sample)
    % Paramètres du régulateur PI
    Ti = 146.07;     % Constante d'intégration
    %Kc = 0.044317;   % Gain proportionnel
    
    % Coefficients de la discrétisation (Tustin)
    % Coefficients du filtre
    num = [0, (1 - exp(-T_sample / Ti))];
    den = [1, -exp(-T_sample / Ti)];
    

    % Application du régulateur sur le signal d'erreur
    u = filter(num, den, entree);  
end

== matlab function Equipe9_Simulateur_Matlab/Conversion resistance//temperature/MATLAB Function ==
  data: u input; y output; R_0 input; T_0 input; B input
function y = fcn(u,R_0,T_0,B) % Fonction non linéaire
% u = R(T) = la valeur de la résistance en fonction de la température (en kelvin)
% y = T = La température de la plaque (en kelvint)



y = 1 ./ ( (1 ./T_0) + (1 ./B) .* log(u ./R_0) );

end
